simulink model "eml_cordic"  (Simulink 7.6)
settings: Solver=FixedStepDiscrete  StartTime=0.0  StopTime=10.0  FixedStep=0.1  RelTol=1e-3
libraries: simulink x2
Description:
  | Embedded MATLAB CORDIC Algorithm for Fixed Point
  | 
  | This model demonstrates how you could implement the CORDIC algorithm for
  | fixed point. The CORDIC algorithm is an interative algorithm to compute the
  | sine/cosine functions by the use of a small lookup table.
  | 
  | The Embedded MATLAB function blocks in this model support code generation with
  | Real-Time Workshop and Real-Time Workshop Embedded Coder.
  | 
  |   Demo Requirements
  | 
  | During this demonstration, Simulink generates code for the simulation in a Simulink
  | project directory created in the current working directory (pwd). If you do not want
  | to affect the current directory (or if you cannot) generate files in this directory, you
  | should change your working directory.
settings Model: Creator=The MathWorks Inc.
settings OptimizationCC: InitFltsAndDblsToZero=on
settings DebuggingCC: SaveWithParameterizedLinksMsg=none  SignalResolutionControl=TryResolveAllWithWarning  MultiTaskDSMMsg=warning  MultiTaskCondExecSysMsg=none  StrictBusMsg=Warning
settings SFSimCC: SFSimEnableDebug=off  SimParseCustomCode=off
settings RTWCC: IncludeERTFirstTime=on
settings GRTTargetCC: TargetFcnLib=ansi_tfl_tmw.mat

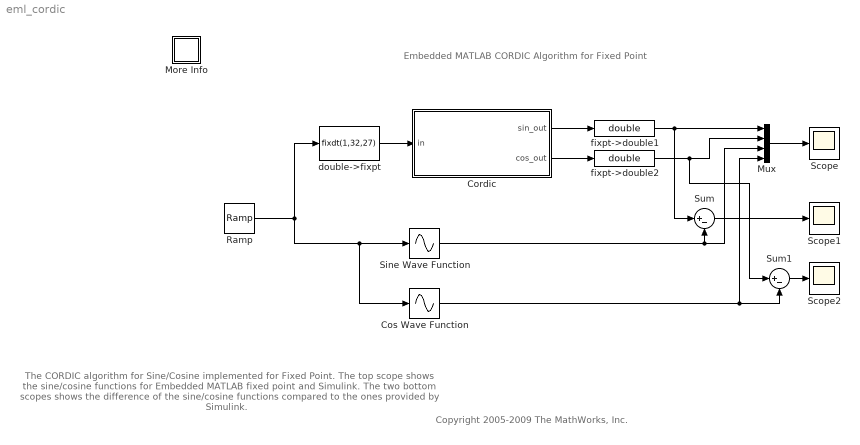
== system eml_cordic ==
  note: Embedded MATLAB CORDIC Algorithm for Fixed Point
  note: The CORDIC algorithm for Sine/Cosine implemented for Fixed Point. The top scope shows
      | the sine/cosine functions for Embedded MATLAB fixed point and Simulink. The two bottom
      | scopes shows the difference of the sine/cosine functions compared to the ones provided by
      | Simulink.
  note: Copyright 2005-2009 The MathWorks, Inc.
  Cordic : Stateflow chart  TreatAsAtomicUnit=on
  Cos Wave Function : Sin  TimeSource=Use external signal  Phase=pi/2  SampleTime=0
  More Info : Subsystem
      mask Display: disp('?')
  Mux : Mux
  Ramp : simulink/Sources/Ramp  SystemSampleTime=-1  slope=1  start=0  X0=0
  Scope : Scope
      settings: YMin=-1.2  YMax=1.2
  Scope1 : Scope
      settings: YMin=-2e-008  YMax=2e-008
  Scope2 : Scope
      settings: YMin=-2e-008  YMax=2e-008  SaveName=ScopeData2
  Sine Wave Function : Sin  TimeSource=Use external signal  SampleTime=0
  Sum : Sum  Inputs=|+-
  Sum1 : Sum  Inputs=|+-
  double->fixpt : DataTypeConversion  OutDataTypeStr=fixdt(1,32,27)
  fixpt->double1 : DataTypeConversion  OutDataTypeStr=double
  fixpt->double2 : DataTypeConversion  OutDataTypeStr=double
  wires:
  Ramp/1 -> double->fixpt/1, Sine Wave Function/1, Cos Wave Function/1
  double->fixpt/1 -> Cordic/1(in)
  Mux/1 -> Scope/1
  Sine Wave Function/1 -> Sum/2, Mux/3
  Cordic/1(sin_out) -> fixpt->double1/1
  fixpt->double1/1 -> Mux/1, Sum/1
  Sum/1 -> Scope1/1
  Cordic/2(cos_out) -> fixpt->double2/1
  fixpt->double2/1 -> Mux/2, Sum1/1
  Cos Wave Function/1 -> Mux/4, Sum1/2
  Sum1/1 -> Scope2/1

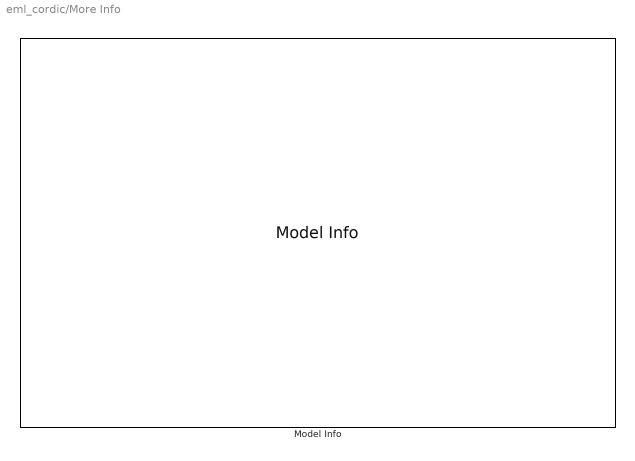
== system eml_cordic/More Info ==
  Model Info : simulink/Model-Wide Utilities/Model Info  SystemSampleTime=-1  InitialBlockCM=None  BlockCM=None  Frame=on  DisplayStringWithTags=|  HorizontalTextAlignment=Left  LeftAlignmentValue=0.02  SourceBlockDiagram=eml_cordic  TagMaxNumber=20
      | Model Description:
      | -------------------
      | 
      | %<Description>

== matlab function Cordic ==
  data: in input double; sin_out output double; cos_out output double
function [sin_out,cos_out]  = cordic_sin_cos(in)
% Test for cordic implementation of sin/cos

wordLength = 32;
fractionLength = 27;

wL = wordLength;
fL = fractionLength;

t = numerictype(1,wordLength,fractionLength);

m = fimath('MaxProductWordLength',wL,'MaxSumWordLength',wL,...
           'ProductMode','SpecifyPrecision',...
           'ProductWordLength',wL,...
           'ProductFractionLength',fL,...
           'SumMode','SpecifyPrecision',...
           'SumWordLength',wL,...
           'SumFractionLength',fL);

%
% fimath is lost so we need to reset it
%

args = fi(in,t,m);

sin_out = args;
cos_out = args;

for i = 1:length(args)
    arg = args(i);
    while arg >= 2*pi
        arg = arg - 2*pi;
    end
    while arg < 0
        arg = arg + 2*pi;
    end
    sin_out(i) = fi_sin(arg);
    cos_out(i) = fi_cos(arg);
end

function y = fi_sin(x)
    if x < pi/2
        [y,t] = fi_sin_cos(x);
    else
        [y0,t] = fi_sin_cos(x-pi);
        y = -y0;
    end
        
function y = fi_cos(x)
    if x < pi/2
        [t,y] = fi_sin_cos(x);
    else
        [t,y0] = fi_sin_cos(x-pi);
        y = -y0;
    end

function [scale,ks,phases] = cordic_table
    wordLength = 31;
    fractionLength = 28;

    wL = wordLength;
    fL = fractionLength;

    m = fimath('MaxProductWordLength',wL,'MaxSumWordLength',wL,...
                'ProductMode','SpecifyPrecision',...
                'ProductWordLength',wL,...
                'ProductFractionLength',fL,...
                'SumMode','SpecifyPrecision',...
                'SumWordLength',wL,...
                'SumFractionLength',fL);
    t = numerictype(1,wL,fL);
    k0 = fi(2^0,t,m);
    p0 = atan(double(k0));
    k1 = fi(2^-1,t,m);
    p1 = atan(double(k1));
    k2 = fi(2^-2,t,m);
    p2 = atan(double(k2));
    k3 = fi(2^-3,t,m);
    p3 = atan(double(k3));
    k4 = fi(2^-4,t,m);
    p4 = atan(double(k4));
    k5 = fi(2^-5,t,m);
    p5 = atan(double(k5));
    k6 = fi(2^-6,t,m);
    p6 = atan(double(k6));
    k7 = fi(2^-7,t,m);
    p7 = atan(double(k7));
    k8 = fi(2^-8,t,m);
    p8 = atan(double(k8));
    k9 = fi(2^-9,t,m);
    p9 = atan(double(k9));
    k10 = fi(2^-10,t,m);
    p10 = atan(double(k10));
    k11 = fi(2^-11,t,m);
    p11 = atan(double(k11));
    k12 = fi(2^-12,t,m);
    p12 = atan(double(k12));
    k13 = fi(2^-13,t,m);
    p13 = atan(double(k13));
    k14 = fi(2^-14,t,m);
    p14 = atan(double(k14));
    k15 = fi(2^-15,t,m);
    p15 = atan(double(k15));
    k16 = fi(2^-16,t,m);
    p16 = atan(double(k16));
    k17 = fi(2^-17,t,m);
    p17 = atan(double(k17));
    k18 = fi(2^-18,t,m);
    p18 = atan(double(k18));
    k19 = fi(2^-19,t,m);
    p19 = atan(double(k19));
    k20 = fi(2^-20,t,m);
    p20 = atan(double(k20));
    k21 = fi(2^-21,t,m);
    p21 = atan(double(k21));
    k22 = fi(2^-22,t,m);
    p22 = atan(double(k22));
    k23 = fi(2^-23,t,m);
    p23 = atan(double(k23));
    k24 = fi(2^-24,t,m);
    p24 = atan(double(k24));
    k25 = fi(2^-25,t,m);
    p25 = atan(double(k25));
    k26 = fi(2^-26,t,m);
    p26 = atan(double(k26));
    k27 = fi(2^-27,t,m);
    p27 = atan(double(k27));
    ks = [k0 k1 k2 k3 k4 k5 k6 k7 k8 k9 k10 k11 k12 k13 k14 k15 k16 k17 k18 k19 k20 k21 k22 k23 k24 k25 k26 k27];
    phases = fi([p0 p1 p2 p3 p4 p5 p6 p7 p8 p9 p10 p11 p12 p13 p14 p15 p16 p17 p18 p19 p20 p21 p22 p23 p24 p25 p26 p27],t,m);

    p = fi(0,t,m);
    z = fi(complex(1,0),t,m);
    for i=1:length(ks)
        if imag(z) >= 0.0
            z = complex(real(z)+imag(z)*ks(i),...
                        imag(z)-real(z)*ks(i));
            p = p + phases(i);
        else
            z = complex(real(z)-imag(z)*ks(i),...
                        imag(z)+real(z)*ks(i));
            p = p - phases(i);
        end
    end
    scale = divide(t,1,real(z));
    
function [sin_x,cos_x] = fi_sin_cos(x)
    [scale,ks,phases] = cordic_table;
    t = numerictype(scale);
    m = fimath(scale);
    p = fi(0,t,m);
    if x > pi/2
        z = fi(complex(0,1),t,m);
        p = fi(pi/2,t,m);
    elseif x < -pi/2
        z = fi(complex(0,-1),t,m);
        p = fi(-pi/2,t,m);
    else
        z = fi(complex(1,0),t,m);
        p = fi(0,t,m);
    end
    for i = 1:length(ks)
        if x < p
            z = complex(real(z)+imag(z)*ks(i),...
                        imag(z)-real(z)*ks(i));
            p = p - phases(i);
        else
            z = complex(real(z)-imag(z)*ks(i),...
                        imag(z)+real(z)*ks(i));
            p = p + phases(i);
        end
    end
    sin_x = fi(imag(z) * scale,numerictype(x),fimath(x));
    cos_x = fi(real(z) * scale,numerictype(x),fimath(x));
